simulink model "EV_EBW2018B"  (Simulink 9.2)
settings: Solver=VariableStepAuto  StartTime=0.0  StopTime=10.0  RelTol=1e-3
InitFcn:
  | run model_par.m
values from neighbouring files (symbols this model uses):
  A = cell2mat(A_cell)    [MPCAPA.m]    (also in model_par.m = [(k1+k2)/m/v (a*k1-b*k2)/m/v/v-1;(a*k1-b*k2)/Iz (a*a*k1+b*b*)
  B = cell2mat(B_cell)    [MPCAPA.m]    (also in model_par.m = [-k1/m/v;-a*k1/Iz])
  C = [1 0 0 0 0;0 1 0 0 0;0 0 1 0 0;]    [MPCAPA.m]    (also in model_par.m = [1 0;0 1])
  Cfm = 0.0014    [model_par.m]
  Cr = 2500    [model_par.m]
  D = [0;0]    [model_par.m]
  ifm = 18    [model_par.m]
  Jfm = 0.00063    [model_par.m]
  kfc = 245    [model_par.m]
  kfe = 0.0031    [model_par.m]
  kft = 0.0417    [model_par.m]
  Lfa = 0.00049    [model_par.m]
  lfl = 0.316    [model_par.m]
  lfr = 0.316    [model_par.m]
  mr = 2.5    [model_par.m]
  Rfa = 0.02    [model_par.m]
  rp = 6.37    [model_par.m]
undefined symbols (not defined in the file or in its folder): sigbuilder_block
libraries: simulink x3, Solver_SF x1
settings Model: Creator=Faith丶Kobe  LastModifiedBy=15044
settings DataIOCC: LimitDataPoints=off  SaveFormat=Dataset  SignalLoggingSaveFormat=Dataset
settings OptimizationCC: LifeSpan=auto
settings DebuggingCC: UnderspecifiedInitializationDetection=Simplified  MergeDetectMultiDrivingBlocksExec=error  FcnCallInpInsideContextMsg=error  StateNameClashWarn=none  SFUnexpectedBacktrackingDiag=error  SFNoUnconditionalDefaultTransitionDiag=error  SFExecutionAtInitializationDiag=warning
settings HardwareCC: ProdBitPerPointer=64  ProdBitPerSizeT=64  ProdBitPerPtrDiffT=64  ProdLargestAtomicFloat=Float  ProdIntDivRoundTo=Zero  ProdEndianess=LittleEndian  ProdWordSize=64  ProdHWDeviceType=Intel->x86-64 (Windows64)
settings ModelReferenceCC: PropagateSignalLabelsOutOfModel=on
settings SFSimCC: SimUseLocalCustomCode=on
settings RTWCC: RTWUseLocalCustomCode=on
settings CodeAppCC: StateflowObjectComments=off
settings GRTTargetCC: TargetLangStandard=C99 (ISO)  GeneratePreprocessorConditionals=Use local settings  CombineOutputUpdateFcns=on  GRTInterface=off
settings ConfigComp: CovMetricSettings=dwe  CovHtmlReporting=off  CovSaveCumulativeToWorkspaceVar=off  CovSaveSingleToWorkspaceVar=off  CovExternalEMLEnable=on

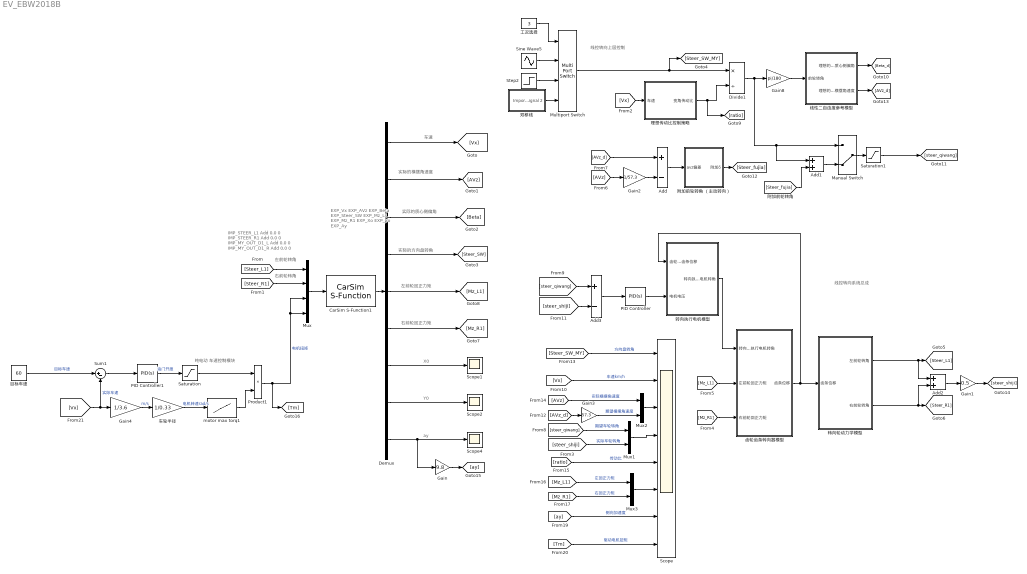
== system EV_EBW2018B ==
  note: IMP_STEER_L1 Add 0.0 0
      | IMP_STEER_R1 Add 0.0 0
      | IMP_MY_OUT_D1_L Add 0.0 0
      | IMP_MY_OUT_D1_R Add 0.0 0
  note: 线控转向系统总成
  note: 线控转向上层控制
  note: 右前轮转角
  note: 左前轮转角
  note: 车速
  note: 左前轮回正力矩
  note: 实际的横摆角速度
  note: 实际的质心侧偏角
  note: 右前轮回正力矩
  note: 实际的方向盘转角
  note: X0
  note: Y0
  note: ay
  note: 纯电动 车速控制模块
  note: EXP_Vx
      | EXP_AVz
      | EXP_Beta
      | EXP_Steer_SW
      | EXP_Mz_L1
      | EXP_Mz_R1
      | EXP_Xo
      | EXP_Yo
      | EXP_Ay
  Add : Sum  Inputs=+-
  Add1 : Sum
  Add2 : Sum
  Add3 : Sum  Inputs=+-
  CarSim S-Function1 : Solver_SF/CarSim S-Function  Priority=1  VehicleCode=i_i  SIMFILE=simfile
  Demux : Demux  Outputs=9
  Divide1 : Product  Inputs=*/
  Gain : Gain  Gain=9.8
  Gain1 : Gain  Gain=0.5
  Gain2 : Gain  Gain=1/57.3
  Gain3 : Gain  Gain=57.3
  Gain4 : Gain  Gain=1/3.6
  Gain8 : Gain  Gain=pi/180
  Manual Switch : ManualSwitch  CurrentSetting=0
  Multiport Switch : MultiPortSwitch
  Mux : Mux
  Mux1 : Mux  Inputs=2
  Mux2 : Mux  Inputs=2
  Mux3 : Mux  Inputs=2
  PID Controller : simulink/Continuous/PID Controller  Controller=PID  Form=Parallel  TimeDomain=Continuous-time  SampleTime=-1  IntegratorMethod=Forward Euler  FilterMethod=Forward Euler  ControllerParametersSource=internal  P=300  I=30  D=10  UseFilter=on  N=100  TunerSelectOption=Transfer Function Based (PID Tuner App)  InitialConditionSource=internal  InitialConditionForIntegrator=0  InitialConditionForFilter=0  DifferentiatorICPrevScaledInput=0  ExternalReset=none  TrackingMode=off  Kt=1  LimitOutput=off  UpperSaturationLimit=inf  LowerSaturationLimit=-inf  LinearizeAsGain=on  AntiWindupMode=none  Kb=1  POutMin=[]  POutMax=[]  IOutMin=[]  IOutMax=[]  DOutMin=[]  DOutMax=[]  NOutMin=[]  NOutMax=[]  SumOutMin=[]  SumOutMax=[]  SaturationOutMin=[]  SaturationOutMax=[]  PParamMin=[]  PParamMax=[]  IParamMin=[]  IParamMax=[]  DParamMin=[]  DParamMax=[]  NParamMin=[]  NParamMax=[]  KbParamMin=[]  KbParamMax=[]  KtParamMin=[]  KtParamMax=[]  KbOutMin=[]  KbOutMax=[]  KtOutMin=[]  KtOutMax=[]  IntegratorOutMin=[]  IntegratorOutMax=[]  FilterOutMin=[]  FilterOutMax=[]  SumI1OutMin=[]  SumI1OutMax=[]  SumI2OutMin=[]  SumI2OutMax=[]  SumI3OutMin=[]  SumI3OutMax=[]  SumI4OutMin=[]  SumI4OutMax=[]  SumDOutMin=[]  SumDOutMax=[]  DifferentiatorOutMin=[]  DifferentiatorOutMax=[]  FilterDiffOutCoefMin=[]  FilterDiffOutCoefMax=[]  ReciprocalOutMin=[]  ReciprocalOutMax=[]  SumDenOutMin=[]  SumDenOutMax=[]  SumNumOutMin=[]  SumNumOutMax=[]  DivideOutMin=[]  DivideOutMax=[]  IntegratorContinuousStateAttributes=''  IntegratorStateMustResolveToSignalObject=off  IntegratorRTWStateStorageClass=Auto  FilterContinuousStateAttributes=''  FilterStateMustResolveToSignalObject=off  FilterRTWStateStorageClass=Auto  ParallelPVariant=InternalParameters  IdealPVariant=Disabled  IVariant=InternalParameters  DVariant=InternalParameters  IntegratorVariant=Continuous  SatVariant=Disabled  AWVariant=Passthrough  PCopyVariant=Disabled  TRVariant=Disabled  FdbkBlocksVariant=Forward  IdealPFdbkVariant=Disabled  SatFdbkVariant=Disabled  DerivativeFilterVariant=ContFilter  NVariant=InternalParameters  NCopyVariant=Disabled  FilterICVariant=InternalICsFilter  IntegratorICVariant=InternalICs  ExternalResetVariant=Disabled  TRSumVariant=Passthrough  SumFdbkVariant=Disabled  SumVariant=Sum_PID
  PID Controller1 : simulink/Continuous/PID Controller  Controller=PID  Form=Parallel  TimeDomain=Continuous-time  SampleTime=-1  IntegratorMethod=Forward Euler  FilterMethod=Forward Euler  ControllerParametersSource=internal  P=1  I=0.5  D=0  UseFilter=on  N=100  TunerSelectOption=Transfer Function Based (PID Tuner App)  InitialConditionSource=internal  InitialConditionForIntegrator=0  InitialConditionForFilter=0  DifferentiatorICPrevScaledInput=0  ExternalReset=none  TrackingMode=off  Kt=1  LimitOutput=off  UpperSaturationLimit=inf  LowerSaturationLimit=-inf  LinearizeAsGain=on  AntiWindupMode=none  Kb=1  POutMin=[]  POutMax=[]  IOutMin=[]  IOutMax=[]  DOutMin=[]  DOutMax=[]  NOutMin=[]  NOutMax=[]  SumOutMin=[]  SumOutMax=[]  SaturationOutMin=[]  SaturationOutMax=[]  PParamMin=[]  PParamMax=[]  IParamMin=[]  IParamMax=[]  DParamMin=[]  DParamMax=[]  NParamMin=[]  NParamMax=[]  KbParamMin=[]  KbParamMax=[]  KtParamMin=[]  KtParamMax=[]  KbOutMin=[]  KbOutMax=[]  KtOutMin=[]  KtOutMax=[]  IntegratorOutMin=[]  IntegratorOutMax=[]  FilterOutMin=[]  FilterOutMax=[]  SumI1OutMin=[]  SumI1OutMax=[]  SumI2OutMin=[]  SumI2OutMax=[]  SumI3OutMin=[]  SumI3OutMax=[]  SumI4OutMin=[]  SumI4OutMax=[]  SumDOutMin=[]  SumDOutMax=[]  DifferentiatorOutMin=[]  DifferentiatorOutMax=[]  FilterDiffOutCoefMin=[]  FilterDiffOutCoefMax=[]  ReciprocalOutMin=[]  ReciprocalOutMax=[]  SumDenOutMin=[]  SumDenOutMax=[]  SumNumOutMin=[]  SumNumOutMax=[]  DivideOutMin=[]  DivideOutMax=[]  IntegratorContinuousStateAttributes=''  IntegratorStateMustResolveToSignalObject=off  IntegratorRTWStateStorageClass=Auto  FilterContinuousStateAttributes=''  FilterStateMustResolveToSignalObject=off  FilterRTWStateStorageClass=Auto  ParallelPVariant=InternalParameters  IdealPVariant=Disabled  IVariant=InternalParameters  DVariant=InternalParameters  IntegratorVariant=Continuous  SatVariant=Disabled  AWVariant=Passthrough  PCopyVariant=Disabled  TRVariant=Disabled  FdbkBlocksVariant=Forward  IdealPFdbkVariant=Disabled  SatFdbkVariant=Disabled  DerivativeFilterVariant=ContFilter  NVariant=InternalParameters  NCopyVariant=Disabled  FilterICVariant=InternalICsFilter  IntegratorICVariant=InternalICs  ExternalResetVariant=Disabled  TRSumVariant=Passthrough  SumFdbkVariant=Disabled  SumVariant=Sum_PID
  Product1 : Product
  Saturation : Saturate  UpperLimit=1  LowerLimit=-1
  Saturation1 : Saturate  UpperLimit=25  LowerLimit=-25
  Scope : Scope  NumInputPorts=8
  Scope1 : Scope
  Scope2 : Scope
  Scope4 : Scope
  Sine Wave5 : Sin  Amplitude=80  Frequency=pi/2  SampleTime=1e-3
  Step2 : Step  After=60  SampleTime=0
  Sum1 : Sum  Inputs=|+-
  motor max torq1 : Lookup_n-D  NumberOfTableDimensions=1  BreakpointsForDimension1=[0 1200 1500 2000 2500 3000 3500 4000 4500 5000 6000 7000 7500]/3*(2*pi)/60  Table=[150 150 150 150 137 112 90 76 65 60 46 42 42 ]*5  RndMeth=Simplest  InputSameDT=on
  双移线 : Subsystem  Tag=STV Subsys  LoadFcn=sigbuilder_block('load');  StartFcn=sigbuilder_block('start');  StopFcn=sigbuilder_block('stop');  ClipboardFcn=sigbuilder_block('clipboard');  mask(Sigbuilder block){tuvar=[0:10]}
      mask help: Simulink:masks:SigbuilderBlock_MD
      mask init:
      | if ~strcmp(get_param(bdroot(gcbh),'SimulationStatus'),'stopped') tuvar = sigbuilder_block('maskInit'); end
      settings: CopyFcn=sigbuilder_block('copy');  DeleteFcn=sigbuilder_block('delete');  ModelCloseFcn=sigbuilder_block('modelClose');  PreSaveFcn=sigbuilder_block('preSave');  PauseFcn=sigbuilder_block('pause');  ContinueFcn=sigbuilder_block('continue');  NameChangeFcn=sigbuilder_block('namechange');  OpenFcn=sigbuilder_block('open',[437.6 199.2 550.4 400 ]);  CloseFcn=sigbuilder_block('close');
      mask Display: plot(0, 0, 100, 100,[2, 2, 32, 32, 2], [68, 8, 8, 68, 68],[32, 2], [38, 38], [32, 19, 2],[53, 60, 44], [32, 17, 17, 2],[16, 16, 31, 31]);txt = getActiveGroup(gcbh);text(2, 100, txt,'verticalAlignment', 'top');
  工况选择 : Constant  Value=3
  理想传动比控制策略 : Subsystem
  目标车速 : Constant  Value=60
  线性二自由度参考模型 : Subsystem
  车轮半径 : Gain  Gain=1/0.33
  转向执行电机模型 : Subsystem
  转向轮动力学模型 : Subsystem
  附加前轮转角 （主动转向） : Subsystem
  齿轮齿条转向器模型 : Subsystem
  wires:
  CarSim S-Function1/1 -> Demux/1
  Demux/2 -> [AVz]
  Demux/5 -> [Mz_L1]
  Demux/6 -> [Mz_R1]
  Demux/4 -> [Steer_SW]
  [Vx] -> 理想传动比控制策略/1(车速)
  齿轮齿条转向器模型/1(齿条位移) -> 转向轮动力学模型/1(齿条位移), 转向执行电机模型/1(齿轮齿条位移)
  理想传动比控制策略/1(变角传动比) -> [ratio], Divide1/2
  Divide1/1 -> Add1/1, Manual Switch/1, Gain8/1
  [Mz_R1] -> 齿轮齿条转向器模型/3(右前轮回正力矩)
  [Mz_L1] -> 齿轮齿条转向器模型/2("左前轮回正力矩 ")
  转向执行电机模型/1(转向执行电机转角) -> 齿轮齿条转向器模型/1(转向执行电机转角)
  Demux/7 -> Scope1/1
  Demux/8 -> Scope2/1
  Demux/9 -> Scope4/1, Gain/1
  [AVz_d] -> Add/1
  Add/1 -> 附加前轮转角 （主动转向）/1(avz偏差)
  Add2/1 -> Gain1/1
  Gain1/1 -> [steer_shiji]
  [steer_qiwang] -> Add3/1
  线性二自由度参考模型/2(理想的横摆角速度) -> [AVz_d]
  Manual Switch/1 -> Saturation1/1
  Add3/1 -> PID Controller/1
  [AVz] -> Gain2/1
  附加前轮转角 （主动转向）/1(附加δ) -> [Steer_fujia]
  Mux/1 -> CarSim S-Function1/1
  转向轮动力学模型/1(左前轮转角) -> Add2/1, [Steer_L1]
  转向轮动力学模型/2(右前轮转角) -> [Steer_R1], Add2/2
  PID Controller/1 -> 转向执行电机模型/2(电机电压)
  Gain8/1 -> 线性二自由度参考模型/1(前轮转角)
  Demux/1 -> [Vx]
  Add1/1 -> Manual Switch/2
  [Steer_fujia] -> Add1/2
  线性二自由度参考模型/1(理想的质心侧偏角) -> [Beta_d]
  [Steer_L1] -> Mux/1
  [Steer_R1] -> Mux/2
  Multiport Switch/1 -> [Steer_SW_MY], Divide1/1
  [steer_shiji] -> Add3/2
  Demux/3 -> [Beta]
  Gain2/1 -> Add/2
  双移线/1(Imported_Signal 2) -> Multiport Switch/4
  Step2/1 -> Multiport Switch/3
  Sine Wave5/1 -> Multiport Switch/2
  工况选择/1 -> Multiport Switch/1
  [steer_shiji] -> Mux1/2  "实际车轮转角"
  [steer_qiwang] -> Mux1/1  "期望车轮转角"
  [Steer_SW_MY] -> Scope/1  "方向盘转角"
  [Vx] -> Scope/2  "车速km/h"
  Mux1/1 -> Scope/4
  [AVz_d] -> Gain3/1
  [AVz] -> Mux2/1  "实际横摆角速度"
  Mux2/1 -> Scope/3
  Gain3/1 -> Mux2/2  "期望横摆角速度"
  [ratio] -> Scope/5  "传动比"
  [Mz_R1] -> Mux3/2  "右回正力矩"
  [Mz_L1] -> Mux3/1  "左回正力矩"
  Mux3/1 -> Scope/6
  [Vx] -> Gain4/1, Sum1/2  "实际车速"
  车轮半径/1 -> motor max torq1/1  "电机转速rad/s"
  Gain4/1 -> 车轮半径/1  "m/s"
  目标车速/1 -> Sum1/1  "目标车速"
  PID Controller1/1 -> Saturation/1  "油门开度"
  Sum1/1 -> PID Controller1/1
  motor max torq1/1 -> Product1/2
  Gain/1 -> [ay]
  [ay] -> Scope/7  "侧向加速度"
  Product1/1 -> [Tm], Mux/4, Mux/3  "电机扭矩"
  Saturation/1 -> Product1/1
  [Tm] -> Scope/8  "驱动电机扭矩"
  Saturation1/1 -> [steer_qiwang]

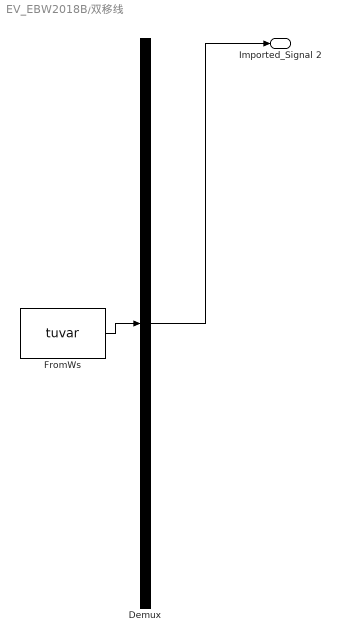
== system EV_EBW2018B/双移线 ==
  Demux : Demux  Tag=STV Demux  Outputs=1
  FromWs : FromWorkspace  Tag=STV FromWs  VariableName=tuvar  SampleTime=0  SigBuilderData=DataTag0  VnvData=DataTag1
      SigBuilderData=|
      | common.afterFinalStr = 'Extrapolate'
      | common.sampleTime = 0
      | dataSet.timeRange = [0 10]
      | dataSet.name = 'Group 1'
      | sbobj.Groups.Name = 'Group 1'
      | sbobj.Groups.Signals.Name = 'Imported_Signal 2'
      | sbobj.Groups.Signals.XData = [0 0.1 0.2 0.3 0.4 0.5 0.6 0.7 0.8 0.9 1 1.1 1.2 1.3 1.4 1.5 1.6 1.7 1.8 1.9 2 2.1 2.2 2.3 2.4 2.5 2.6 2.7 2.8 2.9 3 3.1 3.2 3.3 3.4 3.5 3.6 3.7 3.8 3.9 4 4.1 4.2 4.3 4.4 4.5 4.6 4.7 4.8 4.9 5 5.1 5.2 5.3 5.4 5.5 5.6 5.7 5.8 5.9 6 6.1 6.2 6.3 6.4 6.5 6.6 6.7 6.8 6.9 7 7.1 7.2 7.3 7.4 7.5 7.6 7.7 7.8 7.9 8 8.1 8.2 8.3 8.4 8.5 8.6 8.7 8.8 8.9 9 9.1 9.2 9.3 9.4 9.5 9.6 9.7 9.8 9.9 10]
      | sbobj.Groups.Signals.YData = [0 2e-15 -1e-15 2e-15 3e-15 -4e-15 -7e-15 -1.2e-14 -2.5e-14 -2.6e-14 -2.6e-14 -2.8e-14 -3.1e-14 -2.9e-14 0.00643240194768 0.135992869735 0.714081466198 2.18621253967 4.95506429672 9.06902217865 14.110244751 19.3691310883 23.9145355225 26.7555713654 27.1107311249 24.8026218414 20.1458568573 13.9099187851 6.93898153305 -0.00295856804587 -6.34380245209 -11.6156892776 -15.6708154678 -18.4658203125 -20.0898704529 -20.9298248291 -21.7158126831 -23.2150783539 -25.8503093719 -29.4514636993 -33.2354621887 -36.0566978455 -36.8786582947 -34.9800491333 -30.3304405212 -23.4259147644 -15.2024850845 -6.70892953873 1.36873686314 8.5997838974 14.5263338089 18.986536026 21.893989563 23.2940044403 23.4265060425 22.6326541901 21.1626033783 19.2216682434 16.9881401062 14.6134262085 12.2065095901 9.83658695221 7.57762145996 5.49797391891 3.64690494537 2.04604840279 0.707716107368 -0.364915579557 -1.17712473869 -1.76187896729 -2.14990067482 -2.37109875679 -2.45242214203 -2.42002344131 -2.29916405678 -2.11295723915 -1.88259184361 -1.6265501976 -1.36056053638 -1.09779083729 -0.848720550537 -0.620873212814 -0.418998628855 -0.245289713144 -0.100237056613 0.0174649618566 0.109360992908 0.176871985197 0.22263482213 0.249809131026 0.261431157589 0.260408312082 0.249691009521 0.23174983263 0.20871283114 0.182656258345 0.155265286565 0.127924531698 0.101711906493 0.0774164348841 0.0555743575096]
  Imported_Signal 2 : Outport  Tag=STV Outport
  wires:
  Demux/1 -> Imported_Signal 2/1
  FromWs/1 -> Demux/1

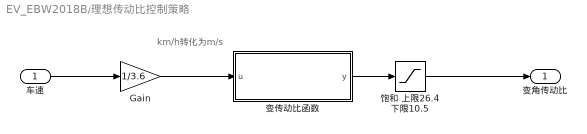
== system EV_EBW2018B/理想传动比控制策略 ==
  note: km/h转化为m/s
  车速 : Inport
  Gain : Gain  Gain=1/3.6
  变传动比函数 : MATLAB Function  TreatAsAtomicUnit=on
  饱和 上限26.4 下限10.5 : Saturate  UpperLimit=26.4  LowerLimit=10.5
  变角传动比 : Outport
  wires:
  车速/1 -> Gain/1
  Gain/1 -> 变传动比函数/1(u)
  变传动比函数/1(y) -> 饱和 上限26.4 下限10.5/1
  饱和 上限26.4 下限10.5/1 -> 变角传动比/1

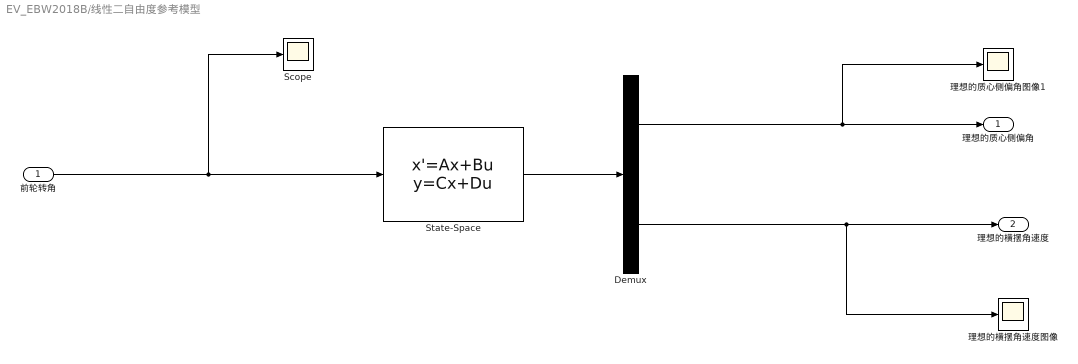
== system EV_EBW2018B/线性二自由度参考模型 ==
  前轮转角 : Inport
  Demux : Demux  Outputs=2
  Scope : Scope
  State-Space : StateSpace  A=A  B=B  C=C  D=D  InitialCondition=0
  理想的横摆角速度图像 : Scope
  理想的质心侧偏角图像1 : Scope
  理想的质心侧偏角 : Outport
  理想的横摆角速度 : Outport  Port=2
  wires:
  前轮转角/1 -> Scope/1, State-Space/1
  State-Space/1 -> Demux/1
  Demux/1 -> 理想的质心侧偏角图像1/1, 理想的质心侧偏角/1
  Demux/2 -> 理想的横摆角速度/1, 理想的横摆角速度图像/1

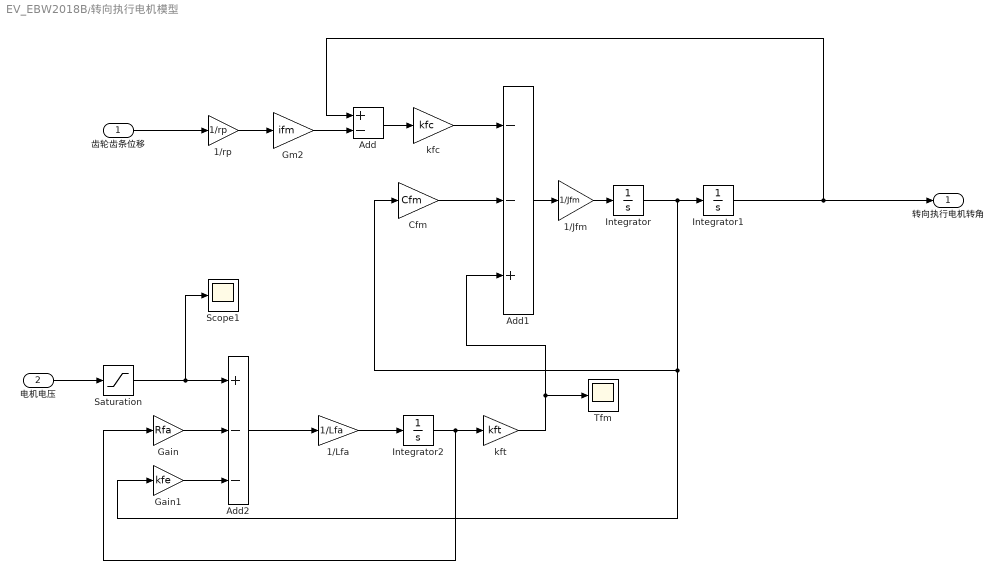
== system EV_EBW2018B/转向执行电机模型 ==
  齿轮齿条位移 : Inport
  电机电压 : Inport  Port=2
  1/Jfm : Gain  Gain=1/Jfm
  1/Lfa : Gain  Gain=1/Lfa
  1/rp : Gain  Gain=1/rp
  Add : Sum  Inputs=+-
  Add1 : Sum  Inputs=--+
  Add2 : Sum  Inputs=+--
  Cfm : Gain  Gain=Cfm
  Gain : Gain  Gain=Rfa
  Gain1 : Gain  Gain=kfe
  Gm2 : Gain  Gain=ifm
  Integrator : Integrator
  Integrator1 : Integrator
  Integrator2 : Integrator
  Saturation : Saturate  UpperLimit=100  LowerLimit=-100
  Scope1 : Scope
  Tfm : Scope
  kfc : Gain  Gain=kfc
  kft : Gain  Gain=kft
  转向执行电机转角 : Outport
  wires:
  齿轮齿条位移/1 -> 1/rp/1
  1/rp/1 -> Gm2/1
  Gm2/1 -> Add/2
  Integrator1/1 -> Add/1, 转向执行电机转角/1
  Add/1 -> kfc/1
  kfc/1 -> Add1/1
  电机电压/1 -> Saturation/1
  Add2/1 -> 1/Lfa/1
  1/Lfa/1 -> Integrator2/1
  Integrator2/1 -> kft/1, Gain/1
  kft/1 -> Add1/3, Tfm/1
  Cfm/1 -> Add1/2
  Gain/1 -> Add2/2
  Gain1/1 -> Add2/3
  Integrator/1 -> Cfm/1, Gain1/1, Integrator1/1
  Add1/1 -> 1/Jfm/1
  1/Jfm/1 -> Integrator/1
  Saturation/1 -> Scope1/1, Add2/1

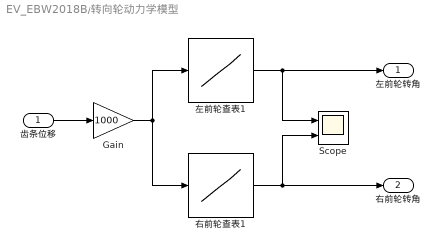
== system EV_EBW2018B/转向轮动力学模型 ==
  齿条位移 : Inport
  Gain : Gain  Gain=1000
  Scope : Scope  NumInputPorts=2
  右前轮查表1 : Lookup_n-D  NumberOfTableDimensions=1  BreakpointsForDimension1=|  Table=|  InternalRulePriority=Speed  RndMeth=Simplest  InputSameDT=on
      BreakpointsForDimension1=|
      | [-68.74666667
      | -66.1025641
      | -63.65432099
      | -61.38095238
      | -59.26436782
      | -57.28888889
      | -55.44086022
      | -53.70833333
      | -52.08080808
      | -50.54901961
      | -49.1047619
      | -47.74074074
      | -46.45045045
      | -45.22807018
      | -44.06837607
      | -42.96666667
      | -41.91869919
      | -40.92063492
      | -39.96899225
      | -39.06060606
      | -38.19259259
      | -37.36231884
      | -36.56737589
      | -35.80555556
      | -35.07482993
      | -34.37333333
      | 0
      | 34.37333333
      | 35.07482993
      | 35.80555556
      | 36.56737589
      | 37.36231884
      | 38.19259259
      | 39.06060606
      | 39.96899225
      | 40.92063492
      | 41.91869919
      | 42.96666667
      | 44.06837607
      | 45.22807018
      | 46.45045045
      | 47.74074074
      | 49.1047619
      | 50.54901961
      | 52.08080808
      | 53.70833333
      | 55.44086022
      | 57.28888889
      | 59.26436782
      | 61.38095238
      | 63.65432099
      | 66.1025641
      | 68.74666667]
      Table=|
      | [-51.70173619
      | -49.01831812
      | -46.60343424
      | -44.4178347
      | -42.42986883
      | -40.61362061
      | -38.94760638
      | -37.41383314
      | -35.99709892
      | -34.68446142
      | -33.46482735
      | -32.32863026
      | -31.26757472
      | -30.27443098
      | -29.34286857
      | -28.46732043
      | -27.64287104
      | -26.86516375
      | -26.13032354
      | -25.4348923
      | -24.77577418
      | -24.15018946
      | -23.55563517
      | -22.98985153
      | -22.45079315
      | -21.93660415
      | 0
      | 17.98751142
      | 18.33767425
      | 18.70226961
      | 19.08225052
      | 19.47866018
      | 19.89264357
      | 20.32546085
      | 20.77850307
      | 21.25331074
      | 21.75159574
      | 22.27526751
      | 22.8264645
      | 23.40759213
      | 24.0213692
      | 24.67088495
      | 25.35966994
      | 26.09178521
      | 26.87193547
      | 27.70561519
      | 28.59929947
      | 29.56069814
      | 30.59910026
      | 31.72585173
      | 32.95503452
      | 34.30446174
      | 35.7971885]
  左前轮查表1 : Lookup_n-D  NumberOfTableDimensions=1  BreakpointsForDimension1=|  Table=|  InternalRulePriority=Speed  RndMeth=Simplest  InputSameDT=on
      BreakpointsForDimension1=|
      | [-68.74666667
      | -66.1025641
      | -63.65432099
      | -61.38095238
      | -59.26436782
      | -57.28888889
      | -55.44086022
      | -53.70833333
      | -52.08080808
      | -50.54901961
      | -49.1047619
      | -47.74074074
      | -46.45045045
      | -45.22807018
      | -44.06837607
      | -42.96666667
      | -41.91869919
      | -40.92063492
      | -39.96899225
      | -39.06060606
      | -38.19259259
      | -37.36231884
      | -36.56737589
      | -35.80555556
      | -35.07482993
      | -34.37333333
      | 0
      | 34.37333333
      | 35.07482993
      | 35.80555556
      | 36.56737589
      | 37.36231884
      | 38.19259259
      | 39.06060606
      | 39.96899225
      | 40.92063492
      | 41.91869919
      | 42.96666667
      | 44.06837607
      | 45.22807018
      | 46.45045045
      | 47.74074074
      | 49.1047619
      | 50.54901961
      | 52.08080808
      | 53.70833333
      | 55.44086022
      | 57.28888889
      | 59.26436782
      | 61.38095238
      | 63.65432099
      | 66.1025641
      | 68.74666667]
      Table=|
      | [-35.7971885
      | -34.30446174
      | -32.95503452
      | -31.72585173
      | -30.59910026
      | -29.56069814
      | -28.59929947
      | -27.70561519
      | -26.87193547
      | -26.09178521
      | -25.35966994
      | -24.67088495
      | -24.0213692
      | -23.40759213
      | -22.8264645
      | -22.27526751
      | -21.75159574
      | -21.25331074
      | -20.77850307
      | -20.32546085
      | -19.89264357
      | -19.47866018
      | -19.08225052
      | -18.70226961
      | -18.33767425
      | -17.98751142
      | 0
      | 21.93660415
      | 22.45079315
      | 22.98985153
      | 23.55563517
      | 24.15018946
      | 24.77577418
      | 25.4348923
      | 26.13032354
      | 26.86516375
      | 27.64287104
      | 28.46732043
      | 29.34286857
      | 30.27443098
      | 31.26757472
      | 32.32863026
      | 33.46482735
      | 34.68446142
      | 35.99709892
      | 37.41383314
      | 38.94760638
      | 40.61362061
      | 42.42986883
      | 44.4178347
      | 46.60343424
      | 49.01831812
      | 51.70173619]
  左前轮转角 : Outport
  右前轮转角 : Outport  Port=2
  wires:
  齿条位移/1 -> Gain/1
  Gain/1 -> 右前轮查表1/1, 左前轮查表1/1
  左前轮查表1/1 -> Scope/1, 左前轮转角/1
  右前轮查表1/1 -> 右前轮转角/1, Scope/2

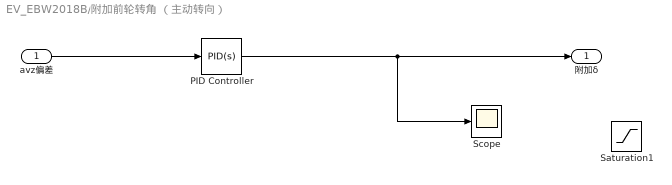
== system EV_EBW2018B/附加前轮转角 （主动转向） ==
  avz偏差 : Inport
  PID Controller : simulink/Continuous/PID Controller  Controller=PID  Form=Parallel  TimeDomain=Continuous-time  SampleTime=-1  IntegratorMethod=Forward Euler  FilterMethod=Forward Euler  ControllerParametersSource=internal  P=50  I=7  D=1  UseFilter=on  N=100  TunerSelectOption=Transfer Function Based (PID Tuner App)  InitialConditionSource=internal  InitialConditionForIntegrator=0  InitialConditionForFilter=0  DifferentiatorICPrevScaledInput=0  ExternalReset=none  TrackingMode=off  Kt=1  LimitOutput=off  UpperSaturationLimit=inf  LowerSaturationLimit=-inf  LinearizeAsGain=on  AntiWindupMode=none  Kb=1  POutMin=[]  POutMax=[]  IOutMin=[]  IOutMax=[]  DOutMin=[]  DOutMax=[]  NOutMin=[]  NOutMax=[]  SumOutMin=[]  SumOutMax=[]  SaturationOutMin=[]  SaturationOutMax=[]  PParamMin=[]  PParamMax=[]  IParamMin=[]  IParamMax=[]  DParamMin=[]  DParamMax=[]  NParamMin=[]  NParamMax=[]  KbParamMin=[]  KbParamMax=[]  KtParamMin=[]  KtParamMax=[]  KbOutMin=[]  KbOutMax=[]  KtOutMin=[]  KtOutMax=[]  IntegratorOutMin=[]  IntegratorOutMax=[]  FilterOutMin=[]  FilterOutMax=[]  SumI1OutMin=[]  SumI1OutMax=[]  SumI2OutMin=[]  SumI2OutMax=[]  SumI3OutMin=[]  SumI3OutMax=[]  SumI4OutMin=[]  SumI4OutMax=[]  SumDOutMin=[]  SumDOutMax=[]  DifferentiatorOutMin=[]  DifferentiatorOutMax=[]  FilterDiffOutCoefMin=[]  FilterDiffOutCoefMax=[]  ReciprocalOutMin=[]  ReciprocalOutMax=[]  SumDenOutMin=[]  SumDenOutMax=[]  SumNumOutMin=[]  SumNumOutMax=[]  DivideOutMin=[]  DivideOutMax=[]  IntegratorContinuousStateAttributes=''  IntegratorStateMustResolveToSignalObject=off  IntegratorRTWStateStorageClass=Auto  FilterContinuousStateAttributes=''  FilterStateMustResolveToSignalObject=off  FilterRTWStateStorageClass=Auto  ParallelPVariant=InternalParameters  IdealPVariant=Disabled  IVariant=InternalParameters  DVariant=InternalParameters  IntegratorVariant=Continuous  SatVariant=Disabled  AWVariant=Passthrough  PCopyVariant=Disabled  TRVariant=Disabled  FdbkBlocksVariant=Forward  IdealPFdbkVariant=Disabled  SatFdbkVariant=Disabled  DerivativeFilterVariant=ContFilter  NVariant=InternalParameters  NCopyVariant=Disabled  FilterICVariant=InternalICsFilter  IntegratorICVariant=InternalICs  ExternalResetVariant=Disabled  TRSumVariant=Passthrough  SumFdbkVariant=Disabled  SumVariant=Sum_PID
  Saturation1 : Saturate  UpperLimit=25  LowerLimit=-25
  Scope : Scope
  附加δ : Outport
  wires:
  avz偏差/1 -> PID Controller/1
  PID Controller/1 -> Scope/1, 附加δ/1

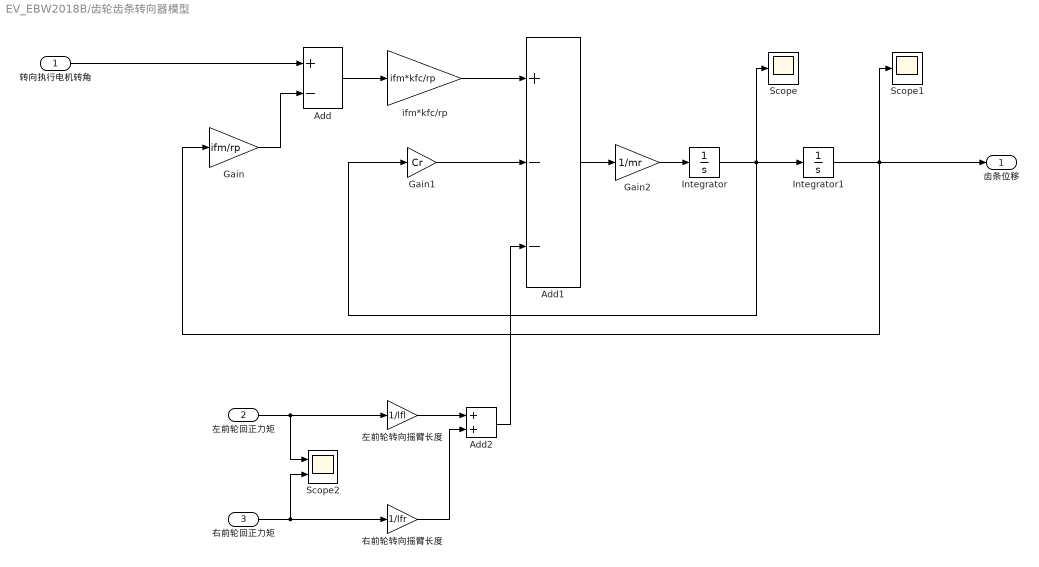
== system EV_EBW2018B/齿轮齿条转向器模型 ==
  转向执行电机转角 : Inport
  "左前轮回正力矩 " : Inport  Port=2
  右前轮回正力矩 : Inport  Port=3
  Add : Sum  Inputs=+-
  Add1 : Sum  Inputs=+--
  Add2 : Sum
  Gain : Gain  Gain=ifm/rp
  Gain1 : Gain  Gain=Cr
  Gain2 : Gain  Gain=1/mr
  Integrator : Integrator
  Integrator1 : Integrator
  Scope : Scope
  Scope1 : Scope
  Scope2 : Scope  NumInputPorts=2
  ifm*kfc/rp : Gain  Gain=ifm*kfc/rp
  右前轮转向摇臂长度 : Gain  Gain=1/lfr
  左前轮转向摇臂长度 : Gain  Gain=1/lfl
  齿条位移 : Outport
  wires:
  转向执行电机转角/1 -> Add/1
  Add/1 -> ifm*kfc/rp/1
  Gain/1 -> Add/2
  ifm*kfc/rp/1 -> Add1/1
  Gain1/1 -> Add1/2
  Integrator/1 -> Gain1/1, Scope/1, Integrator1/1
  Add1/1 -> Gain2/1
  Gain2/1 -> Integrator/1
  Integrator1/1 -> Gain/1, 齿条位移/1, Scope1/1
  "左前轮回正力矩 "/1 -> 左前轮转向摇臂长度/1, Scope2/1
  右前轮回正力矩/1 -> 右前轮转向摇臂长度/1, Scope2/2
  左前轮转向摇臂长度/1 -> Add2/1
  右前轮转向摇臂长度/1 -> Add2/2
  Add2/1 -> Add1/3

== matlab function 理想传动比控制策略/变传动比函数 ==
  data: u input double; y output double
function y = fcn(u)
L=2.578;Gsw=0.3;
m=1274;a=1.016;b=1.562;
k1=-110000;k2=-78000;
K=m*(a/k2-b/k1)/L/L;
y = u/L/Gsw/(1+K*u*u);
